simulink model "TIM"  (R2017b)
settings: Solver=ode45  StartTime=0.0  StopTime=inf  RelTol=1e-3
undefined symbols (not defined in the file): sigbuilder_block
(part 2 of 2)

== matlab function TIM/Baler/AutoCfg_2 Subsystem/CalcTargetAngel ==
  data: SWL input; TargetAngle output
function TargetAngle = fcn(SWL)

  
TargetAngle = 3*SWL;
end

== matlab function TIM/Baler/AutoCfg_2 Subsystem/CalcTargetSpeed/MATLAB Function ==
  data: u input; TargetSpeed output
function TargetSpeed = fcn(u)

  
TargetSpeed = -.10*u+20;
end

== matlab function TIM/Baler/AutoCfg_2 Subsystem/RearDoorControl/CloseRearDoor ==
  data: DoorStatus input; y output; BaleOutSr input
function y = fcn(DoorStatus, BaleOutSr)
if (DoorStatus==1 &&BaleOutSr==1)
y = 0;
else
 y=DoorStatus;
    
end

== matlab function TIM/Baler/AutoCfg_2 Subsystem/RearDoorControl/OpenRearDoorFunction ==
  data: StopSignal input; Y output; BaleSize input; RearObstSr input

function Y = fcn(StopSignal,BaleSize,RearObstSr)

if (StopSignal==1 && BaleSize==2 && RearObstSr==0)
    Y =1;
else
    
    Y=0;
    
end

== matlab function TIM/Baler/SemiAutoCfg Subsystem/CalcTargetSpeed/MATLAB Function ==
  data: u input; TargetSpeed output
function TargetSpeed = fcn(u)

  
TargetSpeed = -.10*u+20;
end

== matlab function TIM/Baler/SemiAutoCfg Subsystem/RearDoorControl/CloseRearDoor ==
  data: DoorStatus input; y output; BaleOutSr input
function y = fcn(DoorStatus, BaleOutSr)
if (DoorStatus==1 &&BaleOutSr==1)
y = 0;
else
 y=DoorStatus;
    
end

== matlab function TIM/Baler/SemiAutoCfg Subsystem/RearDoorControl/OpenRearDoorFunction ==
  data: StopSignal input; Y output; BaleSize input; RearObstSr input

function Y = fcn(StopSignal,BaleSize,RearObstSr)

if (StopSignal==1 && BaleSize==2 && RearObstSr==0)
    Y =1;
else
    
    Y=0;
    
end

== matlab function TIM/Tractor/ManualCfg SubSystem/setStAngle ==
  data: TAngle input; CAngle output
function CAngle = fcn( TAngle )


   CAngle = TAngle; 
end

== matlab function TIM/Tractor/Auto_Cfg SubSystem/setStAngle ==
  data: TAngle input; CAngle output
function CAngle = fcn( TAngle )


   CAngle = TAngle; 
end

== matlab function TIM/Tractor/SemiAuto_Cfg SubSystem/setStAngle ==
  data: TAngle input; CAngle output
function CAngle = fcn( TAngle )


   CAngle = TAngle; 
end
